simulink model "simulation"  (Simulink 7.9)
settings: Solver=ode45  StartTime=0.0  StopTime=Tsim  RelTol=1e-3
values from neighbouring files (symbols this model uses):
  Fsin = 5.5    [script_simulation.m]
  Te = T/M    (= 0.0625)    [script_simulation.m]    (also in traitement_du_signal.m = 3.125e-06)
settings Model: Creator=ahamada  LastModifiedBy=ahamada

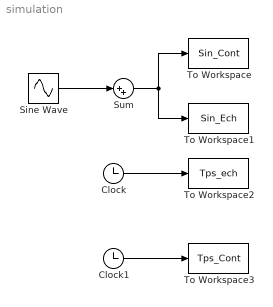
== system simulation ==
  Clock : Clock
  Clock1 : Clock
  Sine Wave : Sin  Frequency=Fsin*2*pi  SampleTime=0
  Sum : Sum  Inputs=|++
  To Workspace : ToWorkspace  VariableName=Sin_Cont  SampleTime=Te/100
  To Workspace1 : ToWorkspace  VariableName=Sin_Ech  SampleTime=Te
  To Workspace2 : ToWorkspace  VariableName=Tps_ech  SampleTime=Te
  To Workspace3 : ToWorkspace  VariableName=Tps_Cont  SampleTime=Te/100
  wires:
  Clock/1 -> To Workspace2/1
  Clock1/1 -> To Workspace3/1
  Sine Wave/1 -> Sum/1
  Sum/1 -> To Workspace/1, To Workspace1/1
